simulink model "lab8"  (Simulink 7.1)
settings: Solver=ode45  StartTime=0.0  StopTime=10  RelTol=1e-3
values from neighbouring files (symbols this model uses):
  den = [1 800 640000]    [lab8.mat]
  K = 2    [lab8.mat]
  num = 640000    [lab8.mat]
  yt1 = 0.2    [lab8.mat]
  yt2 = 1.8    [lab8.mat]
  yt3 = 1.9    [lab8.mat]
  yt4 = 2.1    [lab8.mat]
libraries: simulink x4
settings Model: Creator=ALUNO  LastModifiedBy=ALUNO

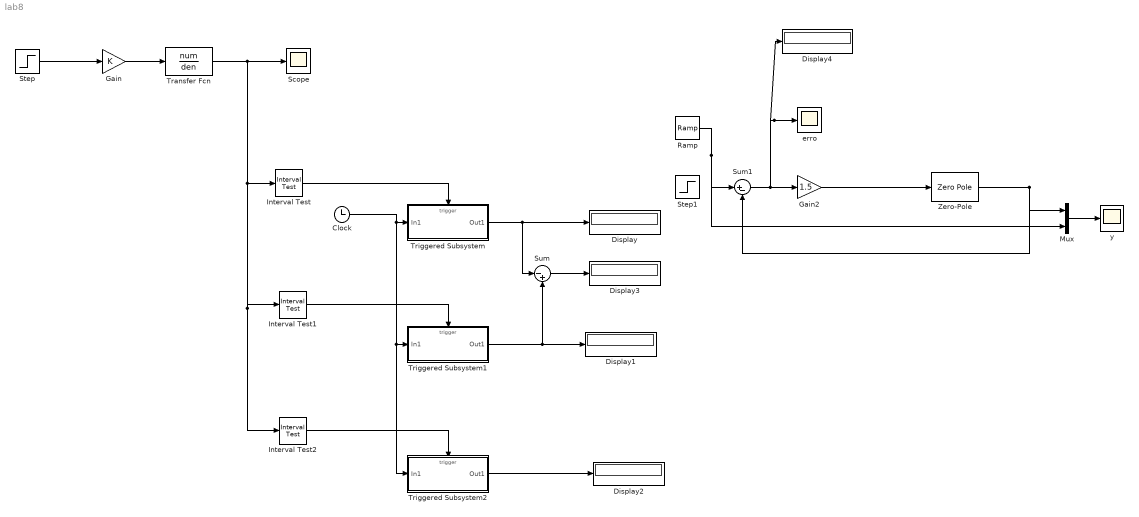
== system lab8 ==
  Clock : Clock
      settings: Decimation=10
  Display{,1..4} (5 alike) : Display
  Gain : Gain  Gain=K  ParameterDataType=sfix(16)  ParameterScaling=2^0  OutDataType=sfix(16)  OutScaling=2^0
  Gain2 : Gain  Gain=1.5  ParameterDataType=sfix(16)  ParameterScaling=2^0  OutDataType=sfix(16)  OutScaling=2^0
  Interval Test : simulink/Logic and Bit Operations/Interval Test  SystemSampleTime=-1  IntervalClosedRight=on  uplimit=yt1  IntervalClosedLeft=on  lowlimit=0  LogicOutDataTypeMode=boolean
  Interval Test1 : simulink/Logic and Bit Operations/Interval Test  SystemSampleTime=-1  IntervalClosedRight=on  uplimit=yt2  IntervalClosedLeft=on  lowlimit=0  LogicOutDataTypeMode=boolean
  Interval Test2 : simulink/Logic and Bit Operations/Interval Test  SystemSampleTime=-1  IntervalClosedRight=on  uplimit=yt4  IntervalClosedLeft=on  lowlimit=yt3  LogicOutDataTypeMode=boolean
  Mux : Mux  Inputs=2
  Ramp : simulink/Sources/Ramp  SystemSampleTime=-1  slope=1  start=0  X0=0
  Scope : Scope
  Step : Step  Time=0  SampleTime=0
  Step1 : Step  SampleTime=0
  Sum : Sum  Inputs=|-+  OutDataType=sfix(16)  OutScaling=2^0
  Sum1 : Sum  Inputs=|+-  OutDataType=sfix(16)  OutScaling=2^0
  Transfer Fcn : TransferFcn  Numerator=num  Denominator=den
  Triggered Subsystem : Subsystem  TreatAsAtomicUnit=on
  Triggered Subsystem1 : Subsystem  TreatAsAtomicUnit=on
  Triggered Subsystem2 : Subsystem  TreatAsAtomicUnit=on
  Zero-Pole : ZeroPole  Zeros=[]  Poles=[-2 -4 0]  Gain=[2]
  erro : Scope
  y : Scope
      settings: SaveName=ScopeData2
  wires:
  Step/1 -> Gain/1
  Gain/1 -> Transfer Fcn/1
  Transfer Fcn/1 -> Scope/1, Interval Test/1, Interval Test2/1, Interval Test1/1
  Interval Test/1 -> Triggered Subsystem/Trigger
  Interval Test1/1 -> Triggered Subsystem1/Trigger
  Interval Test2/1 -> Triggered Subsystem2/Trigger
  Triggered Subsystem/1(Out1) -> Display/1, Sum/1
  Triggered Subsystem1/1(Out1) -> Display1/1, Sum/2
  Triggered Subsystem2/1(Out1) -> Display2/1
  Clock/1 -> Triggered Subsystem/1(In1), Triggered Subsystem2/1(In1), Triggered Subsystem1/1(In1)
  Sum/1 -> Display3/1
  Gain2/1 -> Zero-Pole/1
  Zero-Pole/1 -> Sum1/2, Mux/1
  Sum1/1 -> Gain2/1, erro/1, Display4/1
  Ramp/1 -> Sum1/1, Mux/2
  Mux/1 -> y/1

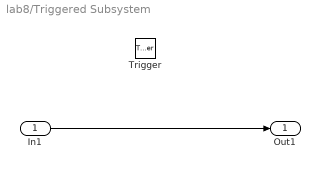
== system lab8/Triggered Subsystem ==
  In1 : Inport  OutDataType=sfix(16)  OutScaling=2^0
  Trigger : TriggerPort  TriggerType=falling
  Out1 : Outport  OutDataType=sfix(16)  OutScaling=2^0
  wires:
  In1/1 -> Out1/1

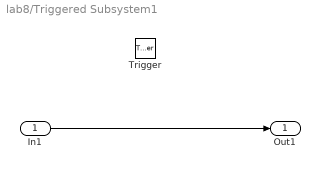
== system lab8/Triggered Subsystem1 ==
  In1 : Inport  OutDataType=sfix(16)  OutScaling=2^0
  Trigger : TriggerPort  TriggerType=falling
  Out1 : Outport  OutDataType=sfix(16)  OutScaling=2^0
  wires:
  In1/1 -> Out1/1

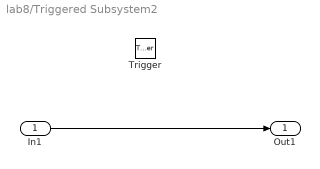
== system lab8/Triggered Subsystem2 ==
  In1 : Inport  OutDataType=sfix(16)  OutScaling=2^0
  Trigger : TriggerPort  TriggerType=either
  Out1 : Outport  OutDataType=sfix(16)  OutScaling=2^0
  wires:
  In1/1 -> Out1/1
